simulink model "roll_loop"  (R2020b)
settings: Solver=VariableStepAuto  StartTime=0.0  StopTime=20  RelTol=1e-3
values from neighbouring files (symbols this model uses):
  Va = uu(4+NN)    [autopilot.m]    (also in true_states.m = uu(1+NN))
undefined symbols (not defined in the file or in its folder): a_beta1, a_beta2, a_phi1, a_phi2, a_theta1, a_theta2, a_theta3, a_V1, a_V2, g, k_d_phi, k_d_theta, k_i_beta, k_i_chi, k_i_h, k_i_V, k_i_V2, k_p_beta, k_p_chi, k_p_h, k_p_phi, k_p_theta, k_p_V, k_p_V2
settings Model: Creator=RunAwayPanda  LastModifiedBy=11814
settings DataIOCC: ReturnWorkspaceOutputs=off
settings DebuggingCC: ArithmeticOperatorsInVariantConditions=warning
settings SFSimCC: SimUseLocalCustomCode=off  CustomCodeUndefinedFunction=UseInterfaceOnly
settings RTWCC: RTWUseLocalCustomCode=off

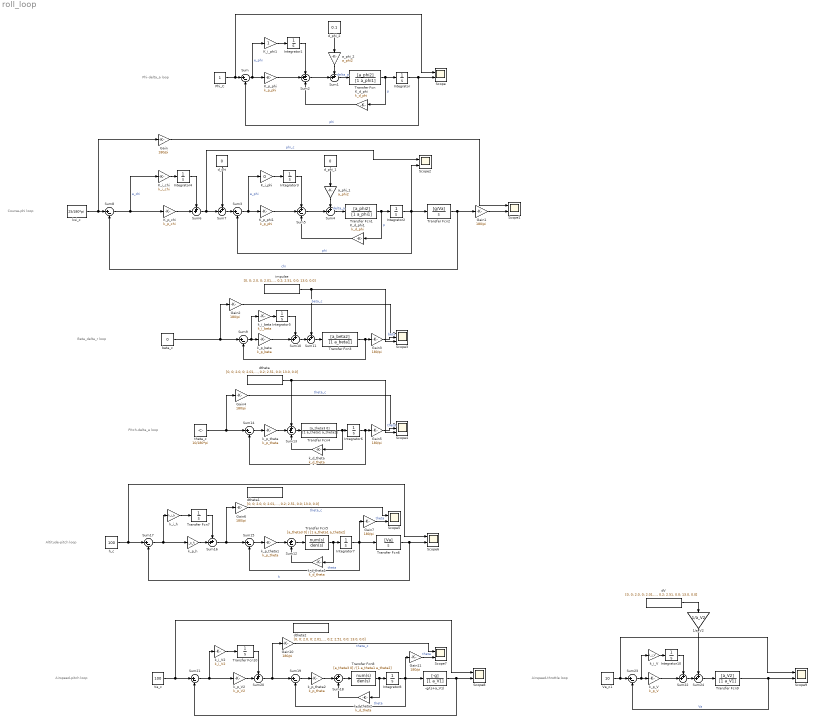
== system roll_loop ==
  note: Airspeed-throttle loop
  note: Airspeed-pitch loop
  note: Altitude-pitch loop
  note: Pitch-delta_e loop
  note: Beta_delta_r loop
  note: Course-phi loop
  note: Phi-delta_a loop
  -g/(s+a_V1) : TransferFcn  Numerator=[-g]  Denominator=[1 a_V1]
  1/a_V2 : Gain  Gain=1/a_V2
  Gain{,1..7,10..11} (10 alike) : Gain  Gain=180/pi
  Integrator{,1..8,10} (10 alike) : Integrator
  K_d_phi : Gain  Gain=k_d_phi
  K_d_phi1 : Gain  Gain=k_d_phi
  K_i_chi : Gain  Gain=k_i_chi
  K_i_phi : Gain  Gain=0
  K_i_phi1 : Gain
  K_p_chi : Gain  Gain=k_p_chi
  K_p_phi : Gain  Gain=k_p_phi
  K_p_phi1 : Gain  Gain=k_p_phi
  Phi_C : Constant
  Scope{,1..2,5..9} (8 alike) : Scope  NumInputPorts=2
  Scope3 : Scope  NumInputPorts=3
  Scope4 : Scope  NumInputPorts=3
  Sum{,3,8..9,14..15,17,19,21,23} (10 alike) : Sum  Inputs=|+-
  Sum{1,4,6..7,10..11,16,20,22,24} (10 alike) : Sum  Inputs=++|
  Sum{2,5,12..13,18} (5 alike) : Sum  Inputs=++-
  Transfer Fcn : TransferFcn  Numerator=[a_phi2]  Denominator=[1 a_phi1]
  Transfer Fcn1 : TransferFcn  Numerator=[a_phi2]  Denominator=[1 a_phi1]
  Transfer Fcn10 : TransferFcn  Denominator=[1 0]
  Transfer Fcn2 : TransferFcn  Numerator=[g/Va]  Denominator=[1 0]
  Transfer Fcn3 : TransferFcn  Numerator=[a_beta2]  Denominator=[1 a_beta1]
  Transfer Fcn4 : TransferFcn  Numerator=[a_theta3 0]  Denominator=[1 a_theta1 a_theta2]
  Transfer Fcn5 : TransferFcn  Numerator=[a_theta3 0]  Denominator=[1 a_theta1 a_theta2]
  Transfer Fcn6 : TransferFcn  Numerator=[Va]  Denominator=[1 0]
  Transfer Fcn7 : TransferFcn  Denominator=[1 0]
  Transfer Fcn8 : TransferFcn  Numerator=[a_theta3 0]  Denominator=[1 a_theta1 a_theta2]
  Transfer Fcn9 : TransferFcn  Numerator=[a_V2]  Denominator=[1 a_V1]
  Va_c : Constant  Value=100
  Va_c1 : Constant  Value=10
  a_phi_1 : Gain  Gain=a_phi2
  a_phi_2 : Gain  Gain=a_phi2
  beta_c : Constant  Value=0
  dV : FromWorkspace  VariableName=[0, 0; 2.0, 0; 2.01, 0.2; 2.5, 0.2; 2.51, 0.0; 13.0, 0.0]
  d_chi : Constant  Value=0
  d_phi_1 : Constant  Value=0
  d_phi_2 : Constant  Value=0.1
  dtheta : FromWorkspace  VariableName=[0, 0; 2.0, 0; 2.01, 0.2; 2.5, 0.2; 2.51, 0.0; 13.0, 0.0]
  dtheta1 : FromWorkspace  VariableName=[0, 0; 2.0, 0; 2.01, 0.2; 2.5, 0.2; 2.51, 0.0; 13.0, 0.0]
  dtheta2 : FromWorkspace  VariableName=[0, 0; 2.0, 0; 2.01, 0.2; 2.5, 0.2; 2.51, 0.0; 13.0, 0.0]
  h_c : Constant  Value=100
  impulse : FromWorkspace  VariableName=[0, 0; 2.0, 0; 2.01, 0.2; 2.5, 0.2; 2.51, 0.0; 13.0, 0.0]
  k_d_theta : Gain  Gain=k_d_theta
  k_d_theta1 : Gain  Gain=k_d_theta
  k_d_theta2 : Gain  Gain=k_d_theta
  k_i_V : Gain  Gain=k_i_V
  k_i_V2 : Gain  Gain=k_i_V2
  k_i_beta : Gain  Gain=k_i_beta
  k_i_h : Gain  Gain=k_i_h
  k_p_V : Gain  Gain=k_p_V
  k_p_V2 : Gain  Gain=k_p_V2
  k_p_beta : Gain  Gain=k_p_beta
  k_p_h : Gain  Gain=k_p_h
  k_p_theta : Gain  Gain=k_p_theta
  k_p_theta1 : Gain  Gain=k_p_theta
  k_p_theta2 : Gain  Gain=k_p_theta
  ksi_c : Constant  Value=25/180*pi
  theta_c : Constant  Value=10/180*pi
  wires:
  Transfer Fcn/1 -> K_d_phi/1, Integrator/1  "p"
  Sum/1 -> K_i_phi1/1, K_p_phi/1  "e_phi"
  Sum1/1 -> Transfer Fcn/1  "delta_a"
  K_d_phi/1 -> Sum2/3
  Integrator/1 -> Scope/2, Sum/2  "phi"
  Phi_C/1 -> Scope/1, Sum/1
  K_i_phi1/1 -> Integrator1/1
  K_p_phi/1 -> Sum2/2
  Sum2/1 -> Sum1/2
  Integrator1/1 -> Sum2/1
  d_phi_2/1 -> a_phi_2/1
  d_phi_1/1 -> a_phi_1/1
  Integrator3/1 -> Sum5/1
  Sum5/1 -> Sum4/2
  K_p_phi1/1 -> Sum5/2
  K_i_phi/1 -> Integrator3/1
  Integrator2/1 -> Scope2/2, Sum3/2, Transfer Fcn2/1  "phi"
  K_d_phi1/1 -> Sum5/3
  Sum4/1 -> Transfer Fcn1/1  "delta_a"
  Sum3/1 -> K_p_phi1/1, K_i_phi/1  "e_phi"
  Transfer Fcn1/1 -> Integrator2/1, K_d_phi1/1  "p"
  Sum8/1 -> K_i_chi/1, K_p_chi/1  "e_chi"
  K_i_chi/1 -> Integrator4/1
  Transfer Fcn2/1 -> Gain1/1, Sum8/2  "chi"
  Integrator4/1 -> Sum6/1
  K_p_chi/1 -> Sum6/2
  Sum6/1 -> Scope2/1, Sum7/2  "phi_c"
  Sum7/1 -> Sum3/1
  d_chi/1 -> Sum7/1
  ksi_c/1 -> Gain/1, Sum8/1
  a_phi_1/1 -> Sum4/1
  a_phi_2/1 -> Sum1/1
  Gain/1 -> Scope1/1
  Gain1/1 -> Scope1/2
  Transfer Fcn3/1 -> Sum9/2, Gain3/1
  beta_c/1 -> Sum9/1, Gain2/1
  Sum9/1 -> k_i_beta/1, k_p_beta/1
  k_i_beta/1 -> Integrator5/1
  k_p_beta/1 -> Sum10/2
  Integrator5/1 -> Sum10/1
  Gain3/1 -> Scope3/2  "beta"
  Gain2/1 -> Scope3/1  "beta_c"
  Sum10/1 -> Sum11/2
  Sum11/1 -> Transfer Fcn3/1
  impulse/1 -> Sum11/1, Scope3/3
  Gain4/1 -> Scope4/1  "theta_c"
  k_p_theta/1 -> Sum13/2
  Transfer Fcn4/1 -> Integrator6/1, k_d_theta/1
  Sum13/1 -> Transfer Fcn4/1
  Gain5/1 -> Scope4/2  "theta"
  Sum14/1 -> k_p_theta/1
  theta_c/1 -> Sum14/1, Gain4/1
  k_d_theta/1 -> Sum13/3
  Integrator6/1 -> Sum14/2, Gain5/1
  k_d_theta1/1 -> Sum12/3
  k_p_theta1/1 -> Sum12/2
  Sum15/1 -> k_p_theta1/1
  Sum16/1 -> Sum15/1, Gain6/1
  Integrator7/1 -> Gain7/1, Transfer Fcn6/1, Sum15/2  "theta"
  Transfer Fcn5/1 -> Integrator7/1, k_d_theta1/1
  Sum12/1 -> Transfer Fcn5/1
  Gain6/1 -> Scope5/1  "theta_c"
  Gain7/1 -> Scope5/2  "theta"
  k_i_h/1 -> Transfer Fcn7/1
  k_p_h/1 -> Sum16/2
  Transfer Fcn7/1 -> Sum16/1
  Sum17/1 -> k_i_h/1, k_p_h/1
  Transfer Fcn6/1 -> Scope6/2, Sum17/2  "h"
  h_c/1 -> Scope6/1, Sum17/1
  -g/(s+a_V1)/1 -> Scope8/2, Sum21/2
  Transfer Fcn10/1 -> Sum20/1
  Sum21/1 -> k_i_V2/1, k_p_V2/1
  k_p_theta2/1 -> Sum18/2
  Sum20/1 -> Sum19/1, Gain10/1
  k_i_V2/1 -> Transfer Fcn10/1
  Gain11/1 -> Scope7/2  "theta"
  k_p_V2/1 -> Sum20/2
  Va_c/1 -> Scope8/1, Sum21/1
  Sum19/1 -> k_p_theta2/1
  Gain10/1 -> Scope7/1  "theta_c"
  Transfer Fcn8/1 -> Integrator8/1, k_d_theta2/1
  Integrator8/1 -> Gain11/1, -g/(s+a_V1)/1, Sum19/2  "theta"
  Sum18/1 -> Transfer Fcn8/1
  k_d_theta2/1 -> Sum18/3
  Va_c1/1 -> Scope9/1, Sum23/1
  Transfer Fcn9/1 -> Sum23/2, Scope9/2  "Va"
  Sum23/1 -> k_i_V/1, k_p_V/1
  k_p_V/1 -> Sum22/2
  k_i_V/1 -> Integrator10/1
  Integrator10/1 -> Sum22/1
  Sum22/1 -> Sum24/2
  Sum24/1 -> Transfer Fcn9/1
  dV/1 -> 1/a_V2/1
  1/a_V2/1 -> Sum24/1
  dtheta/1 -> Sum13/1, Scope4/3
